simulink model "Q2_2"  (R2018b)
settings: Solver=VariableStepAuto  StartTime=0.0  StopTime=10.0  RelTol=1e-3
settings Model: Creator=N.GH  LastModifiedBy=N.GH

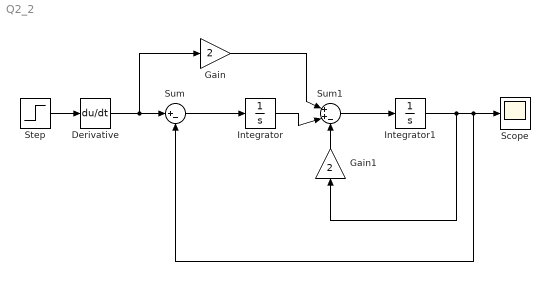
== system Q2_2 ==
  Derivative : Derivative
  Gain : Gain  Gain=2
  Gain1 : Gain  Gain=2
  Integrator : Integrator
  Integrator1 : Integrator
  Scope : Scope
  Step : Step  SampleTime=0
  Sum : Sum  Inputs=|+-
  Sum1 : Sum  Inputs=|++-
  wires:
  Step/1 -> Derivative/1
  Derivative/1 -> Gain/1, Sum/1
  Sum/1 -> Integrator/1
  Sum1/1 -> Integrator1/1
  Integrator1/1 -> Gain1/1, Sum/2, Scope/1
  Gain/1 -> Sum1/1
  Integrator/1 -> Sum1/2
  Gain1/1 -> Sum1/3
